simulink model "Li-ion_battery_vehicle"  (R2021a)
settings: Solver=VariableStepAuto  StartTime=0.0  StopTime=200  RelTol=1e-3
values from neighbouring files (symbols this model uses):
  air_density = 1.225    [matlabnew.mat]
  area = 5    [matlabnew.mat]
  braking_torque_to_pedal_force_ratio = -4    [matlabnew.mat]
  C1_LUT = [1913.6 4625.7 23306 10736 18036 12251 9022.9 12447 18872 40764 18721 33630 ... (21 elements, 7x3)]    [matlabnew.mat]
  Capacity_LUT = [28.0081 27.625 27.6392]    [matlabnew.mat]
  cell_Cp_heat = 810.5328    [matlabnew.mat]
  cell_mass = 1    [matlabnew.mat]
  drag_coefficient = 0.25    [matlabnew.mat]
  dt = 0.01    [matlabnew.mat]
  Em_LUT = [3.4966 3.5519 3.6183 3.7066 3.9131 4.0748 4.1923 3.5057 3.566 3.6337 3.7127 3.9259 ... (21 elements, 7x3)]    [matlabnew.mat]
  force_max_pedal = 500    [matlabnew.mat]
  gear_ratio = 6    [matlabnew.mat]
  gravity = 9.81    [matlabnew.mat]
  max_power = 50000    [matlabnew.mat]
  max_torque = 220    [matlabnew.mat]
  Qe_init = 15.6845    [matlabnew.mat]
  R0_LUT = [0.0117 0.011 0.0114 0.0107 0.0107 0.0113 0.0116 0.0085 0.0085 0.0087 0.0082 0.0083 ... (21 elements, 7x3)]    [matlabnew.mat]
  R1_LUT = [0.0109 0.0069 0.0047 0.0034 0.0033 0.0033 0.0028 0.0029 0.0024 0.0026 0.0016 0.0023 ... (21 elements, 7x3)]    [matlabnew.mat]
  rolling_res_ratio = 0.015    [matlabnew.mat]
  SOC_LUT = [0 0.1 0.25 0.5 0.75 0.9 1]    [matlabnew.mat]
  T_init = 293.15    [matlabnew.mat]
  Temperature_LUT = [278.15 293.15 313.15]    [matlabnew.mat]
  vehicle_mass = 1800    [matlabnew.mat]
  wheel_radius = 0.025    [matlabnew.mat]
undefined symbols (not defined in the file or in its folder): DiscIntNeverNeededParam, sigbuilder_block
libraries: fl_lib x57, fl_ps_legacy_lib x36, nesl_utility x13, LiBatteryElements_lib x4, ee_lib x2, simulink x2, simulink_extras x1, sim3dcameralib x1, sim3dlib x1, sim3dautolib x1
(part 2 of 2)

== system Li-ion_battery_vehicle/Vehicle Control/Max Power ==
  Vspd : Inport
  Abs : Abs
  Constant : Constant
  Math Function : Math  Operator=reciprocal  SignedPower=on  SaturateOnIntegerOverflow=on
  Prevent divide by zero : Switch  Criteria=u2 > Threshold  Threshold=1
  max_power : Gain  Gain=max_power
  Max Power : Outport  VectorParamsAs1DForOutWhenUnconnected=off
  wires:
  Prevent divide by zero/1 -> Math Function/1
  Constant/1 -> Prevent divide by zero/3
  Abs/1 -> Prevent divide by zero/2, Prevent divide by zero/1
  Math Function/1 -> max_power/1
  max_power/1 -> Max Power/1
  Vspd/1 -> Abs/1

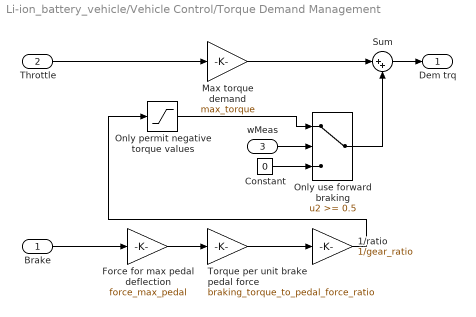
== system Li-ion_battery_vehicle/Vehicle Control/Torque Demand Management ==
  Brake : Inport
  Throttle : Inport  Port=2
  wMeas : Inport  Port=3
  1/ratio : Gain  Gain=1/gear_ratio
  Constant : Constant  Value=0  SampleTime=dt
  Force for max pedal deflection : Gain  Gain=force_max_pedal
  Max torque demand : Gain  Gain=max_torque
  Only permit negative torque values : Saturate  UpperLimit=-10  LowerLimit=-max_torque
  Only use forward braking : Switch  Threshold=0.5  InputSameDT=on
  Sum : Sum  Inputs=|++
  Torque per unit brake pedal force : Gain  Gain=braking_torque_to_pedal_force_ratio
  Dem trq : Outport  VectorParamsAs1DForOutWhenUnconnected=off
  wires:
  Max torque demand/1 -> Sum/1
  Brake/1 -> Force for max pedal deflection/1
  Sum/1 -> Dem trq/1
  Throttle/1 -> Max torque demand/1
  Torque per unit brake pedal force/1 -> 1/ratio/1
  1/ratio/1 -> Only permit negative torque values/1
  Force for max pedal deflection/1 -> Torque per unit brake pedal force/1
  wMeas/1 -> Only use forward braking/2
  Only use forward braking/1 -> Sum/2
  Constant/1 -> Only use forward braking/3
  Only permit negative torque values/1 -> Only use forward braking/1

== system Li-ion_battery_vehicle/Vehicle Control/regenerative braking  ==
  Inclin. : Inport
  " M " : Gain  Gain=vehicle_mass
  1/ratio : Gain  Gain=1/gear_ratio
  Wheel radius : Gain  Gain=wheel_radius
  Feedfwd trq : Outport  VectorParamsAs1DForOutWhenUnconnected=off
  wires:
  Inclin./1 -> " M "/1
  " M "/1 -> Wheel radius/1
  Wheel radius/1 -> 1/ratio/1  "Wheel torque"
  1/ratio/1 -> Feedfwd trq/1  "Motor torque"

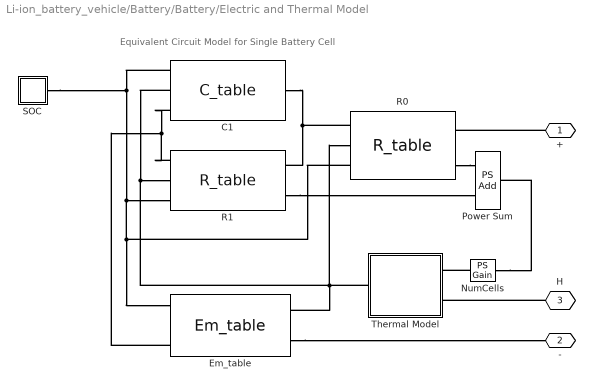
== system Li-ion_battery_vehicle/Battery/Battery/Electric and Thermal Model ==
  note: Equivalent Circuit Model for Single Battery Cell
  " SOC " : Subsystem
  C1 : LiBatteryElements_lib/C_table  C_Table=C1_LUT*Nparallel F  SOC_Table=SOC_LUT  Temp_Table=Temperature_LUT K  v0=0 V
      settings: SourceProductBaseCode=SS  InternalSimscapePortConfiguration="{\"Bottom\":[],\"Left\":[{\"id\":\"p\",\"label\":\"+\",\"type\":\"foundation.electrical.electrical\"},{\"id\":\"T\",\"label\":\"T\",\"type\":\"input\"},{\"id\":\"SOC\",\"label\":\"SOC\",\"type\":\"input\"}],\"Right\":[{\"id\":\"n\",\"label\":\"-\",\"type\":\"foundation.electrical.electrical\"}],\"Top\":[]}"
  Em_table : LiBatteryElements_lib/Em_table  C_Table=Capacity_LUT*Nparallel hr*A  Em_Table=Em_LUT V  SOC_Table=SOC_LUT  Temp_Table=Temperature_LUT K  Qinit=Qe_init*Nparallel hr*A
      settings: SourceProductBaseCode=SS  InternalSimscapePortConfiguration="{\"Bottom\":[],\"Left\":[{\"id\":\"p\",\"label\":\"+\",\"type\":\"foundation.electrical.electrical\"},{\"id\":\"C\",\"label\":\"C\",\"type\":\"output\"},{\"id\":\"SOC\",\"label\":\"SOC\",\"type\":\"output\"}],\"Right\":[{\"id\":\"n\",\"label\":\"-\",\"type\":\"foundation.electrical.electrical\"},{\"id\":\"T\",\"label\":\"T\",\"type\":\"input\"}],\"Top\":[]}"
  NumCells : fl_ps_legacy_lib/Legacy Physical Signals/Functions/PS Gain  gain=Nseries
  Power Sum : fl_ps_legacy_lib/Legacy Physical Signals/Functions/PS Add
      settings: SourceProductBaseCode=SS  InternalSimscapePortConfiguration="{\"Bottom\":[],\"Left\":[{\"id\":\"I1\",\"label\":\"\",\"type\":\"input\"},{\"id\":\"I2\",\"label\":\"\",\"type\":\"input\"}],\"Right\":[{\"id\":\"O\",\"label\":\"\",\"type\":\"output\"}],\"Top\":[]}"
  R0 : LiBatteryElements_lib/R_table  R_Table=R0_LUT/Nparallel Ohm  SOC_Table=SOC_LUT  Temp_Table=Temperature_LUT K
      settings: SourceProductBaseCode=SS  InternalSimscapePortConfiguration="{\"Bottom\":[],\"Left\":[{\"id\":\"p\",\"label\":\"+\",\"type\":\"foundation.electrical.electrical\"},{\"id\":\"T\",\"label\":\"T\",\"type\":\"input\"},{\"id\":\"SOC\",\"label\":\"SOC\",\"type\":\"input\"}],\"Right\":[{\"id\":\"n\",\"label\":\"-\",\"type\":\"foundation.electrical.electrical\"},{\"id\":\"pow\",\"label\":\"POW\",\"type\":\"output\"}],\"Top\":[]}"
  R1 : LiBatteryElements_lib/R_table  R_Table=R1_LUT/Nparallel Ohm  SOC_Table=SOC_LUT  Temp_Table=Temperature_LUT K
      settings: SourceProductBaseCode=SS  InternalSimscapePortConfiguration="{\"Bottom\":[],\"Left\":[{\"id\":\"p\",\"label\":\"+\",\"type\":\"foundation.electrical.electrical\"},{\"id\":\"T\",\"label\":\"T\",\"type\":\"input\"},{\"id\":\"SOC\",\"label\":\"SOC\",\"type\":\"input\"}],\"Right\":[{\"id\":\"n\",\"label\":\"-\",\"type\":\"foundation.electrical.electrical\"},{\"id\":\"pow\",\"label\":\"POW\",\"type\":\"output\"}],\"Top\":[]}"
  Thermal Model : Subsystem
  + : PMIOPort  Side=Right
  - : PMIOPort  Port=2  Side=Right
  H : PMIOPort  Tag=PMCPort  Port=3  Side=Left
  connections:
  NumCells/LConn1 -- Power Sum/RConn1
  +/RConn1 -- R0/RConn1
  C1/LConn2 -- Thermal Model/RConn1 -- Em_table/RConn2 -- R0/LConn2 -- R1/LConn2
  Em_table/LConn1 -- R1/LConn1 -- C1/LConn1
  R1/RConn2 -- Power Sum/LConn2
  R0/RConn2 -- Power Sum/LConn1
  C1/RConn1 -- R1/RConn1 -- R0/LConn1
  Em_table/RConn1 -- -/RConn1
  R0/LConn3 -- Em_table/LConn3 -- " SOC "/LConn1 -- C1/LConn3 -- R1/LConn3
  NumCells/RConn1 -- Thermal Model/LConn1
  H/RConn1 -- Thermal Model/LConn2

== system Li-ion_battery_vehicle/Battery/Cooling System/Heat Exch. Characteristic ==
  Characteristic : Subsystem
  Heat Flow Source : fl_lib/Thermal/Thermal Sources/Controlled Heat Flow Rate Source
  Mass Flow Rate & Thermal Flux Sensor (TL) : fl_lib/Thermal Liquid/Sensors/Mass & Energy Flow Rate Sensor (TL)
      settings: SourceProductBaseCode=SS  InternalSimscapePortConfiguration="{\"Bottom\":[],\"Left\":[{\"id\":\"A\",\"label\":\"A\",\"type\":\"foundation.thermal_liquid.thermal_liquid\"}],\"Right\":[{\"id\":\"B\",\"label\":\"B\",\"type\":\"foundation.thermal_liquid.thermal_liquid\"},{\"id\":\"M\",\"label\":\"M\",\"type\":\"output\"},{\"id\":\"PHI\",\"label\":\"Phi\",\"type\":\"output\"}],\"Top\":[]}"
  Temperature Sensor : fl_lib/Thermal/Thermal Sensors/Temperature Sensor
  ThRef : fl_lib/Thermal/Thermal Elements/Thermal Reference
  Henv : PMIOPort  Side=Right
  Hp : PMIOPort  Port=2  Side=Left
  B : PMIOPort  Port=3  Side=Right
  Phi : PMIOPort  Port=4  Side=Right
  A : PMIOPort  Port=5  Side=Left
  T in : PMIOPort  Port=6  Side=Left
  connections:
  A/RConn1 -- Mass Flow Rate & Thermal Flux Sensor (TL)/LConn1
  Temperature Sensor/LConn1 -- Henv/RConn1 -- Heat Flow Source/RConn2
  ThRef/LConn1 -- Temperature Sensor/RConn1
  Heat Flow Source/LConn1 -- Hp/RConn1
  Mass Flow Rate & Thermal Flux Sensor (TL)/RConn1 -- B/RConn1
  Mass Flow Rate & Thermal Flux Sensor (TL)/RConn3 -- Phi/RConn1
  Mass Flow Rate & Thermal Flux Sensor (TL)/RConn2 -- Characteristic/RConn1
  T in/RConn1 -- Characteristic/RConn2
  Temperature Sensor/RConn2 -- Characteristic/RConn3
  Characteristic/LConn1 -- Heat Flow Source/RConn1

== system Li-ion_battery_vehicle/Battery/Cooling System/Sensing Temperature ==
  Pressure & Temperature Sensor (TL) : fl_lib/Thermal Liquid/Sensors/Pressure & Temperature Sensor (TL)
      settings: SourceProductBaseCode=SS  InternalSimscapePortConfiguration="{\"Bottom\":[],\"Left\":[{\"id\":\"A\",\"label\":\"A\",\"type\":\"foundation.thermal_liquid.thermal_liquid\"}],\"Right\":[{\"id\":\"B\",\"label\":\"B\",\"type\":\"foundation.thermal_liquid.thermal_liquid\"},{\"id\":\"P\",\"label\":\"P\",\"type\":\"output\"},{\"id\":\"T\",\"label\":\"T\",\"type\":\"output\"}],\"Top\":[]}"
  TLRef : fl_lib/Thermal Liquid/Elements/Absolute Reference (TL)
      settings: SourceProductBaseCode=SS
  T : PMIOPort  Side=Right
  A : PMIOPort  Port=2  Side=Left
  connections:
  Pressure & Temperature Sensor (TL)/RConn3 -- T/RConn1
  TLRef/LConn1 -- Pressure & Temperature Sensor (TL)/RConn1
  A/RConn1 -- Pressure & Temperature Sensor (TL)/LConn1

== system Li-ion_battery_vehicle/Battery/DC-DC Converter/Sensing Battery Quantities ==
  Battery Voltage : nesl_utility/PS-Simulink Converter  PhysicalDomain=network_engine_domain  SubClassName=ps_output  LeftPortType=input  RightPortType=output  PseudoPeriodic=off  Frequencies=[]  Unit=V  AffineConversion=off
      settings: SourceProductBaseCode=PW,SS
  Current Sensor : fl_lib/Electrical/Electrical Sensors/Current Sensor
  PS-Simulink Converter1 : nesl_utility/PS-Simulink Converter  PhysicalDomain=network_engine_domain  SubClassName=ps_output  LeftPortType=input  RightPortType=output  PseudoPeriodic=off  Frequencies=[]  Unit=A  AffineConversion=off
      settings: SourceProductBaseCode=PW,SS
  Voltage Sensor : fl_lib/Electrical/Electrical Sensors/Voltage Sensor
  +1 : PMIOPort  Side=Right
  - : PMIOPort  Port=2  Side=Left
  +2 : PMIOPort  Port=3  Side=Right
  tag scope: iBat=global, vBat=global
  wires:
  Battery Voltage/1 -> [vBat]
  PS-Simulink Converter1/1 -> [iBat]
  connections:
  Voltage Sensor/RConn2 -- -/RConn1
  Voltage Sensor/LConn1 -- Current Sensor/LConn1 -- +1/RConn1
  Voltage Sensor/RConn1 -- Battery Voltage/LConn1
  Current Sensor/RConn2 -- +2/RConn1
  Current Sensor/RConn1 -- PS-Simulink Converter1/LConn1

== system Li-ion_battery_vehicle/PMSM Drive/Heat Exch. Characteristic/Characteristic ==
  PS Product : fl_ps_legacy_lib/Legacy Physical Signals/Functions/PS Product
      settings: SourceProductBaseCode=SS
  PS Subtract : fl_ps_legacy_lib/Legacy Physical Signals/Functions/PS Subtract
      settings: SourceProductBaseCode=SS
  Specific dissipation (J/s/K) : fl_ps_legacy_lib/Legacy Physical Signals/Lookup Tables/PS Lookup Table (1D)  x="[0 0.2 0.4  0.7  1 1.2  1.4  2.5 ]"  f=100 * [0 0.5 0.75 0.92 1 1.02 1.03 1.04]  interp_method=1  extrap_method=1
      settings: SourceProductBaseCode=SS  InternalSimscapePortConfiguration="{\"Bottom\":[],\"Left\":[{\"id\":\"I\",\"label\":\"x\",\"type\":\"input\"}],\"Right\":[{\"id\":\"O\",\"label\":\"f\",\"type\":\"output\"}],\"Top\":[]}"
  Specific dissipation (J/s/K) per unit mass flow rate : fl_ps_legacy_lib/Legacy Physical Signals/Functions/PS Gain  gain=100
  Mass Flow : PMIOPort  Side=Left
  Temp Inlet : PMIOPort  Port=2  Side=Left
  Temp Motor : PMIOPort  Port=3  Side=Left
  Q : PMIOPort  Port=4  Side=Right
  connections:
  PS Subtract/RConn1 -- PS Product/LConn1
  Specific dissipation (J/s/K)/RConn1 -- PS Product/LConn2
  Temp Motor/RConn1 -- PS Subtract/LConn1
  PS Subtract/LConn2 -- Temp Inlet/RConn1
  PS Product/RConn1 -- Q/RConn1
  Mass Flow/RConn1 -- Specific dissipation (J/s/K) per unit mass flow rate/LConn1
  Specific dissipation (J/s/K) per unit mass flow rate/RConn1 -- Specific dissipation (J/s/K)/LConn1

== system Li-ion_battery_vehicle/Vehicle Dynamics/Brake Torque/Smooth Sign ==
  1 : fl_lib/Physical Signals/Sources/PS Constant  constant=1
  2 : fl_ps_legacy_lib/Legacy Physical Signals/Functions/PS Gain  gain=2
  exp(2x) : fl_ps_legacy_lib/Legacy Physical Signals/Functions/PS Math Function  fcn_choice=3
      settings: SourceProductBaseCode=SS  InternalSimscapePortConfiguration="{\"Bottom\":[],\"Left\":[{\"id\":\"I\",\"label\":\"\",\"type\":\"input\"}],\"Right\":[{\"id\":\"O\",\"label\":\"\",\"type\":\"output\"}],\"Top\":[]}"
  exp(2x)+1 : fl_ps_legacy_lib/Legacy Physical Signals/Functions/PS Add
      settings: SourceProductBaseCode=SS  InternalSimscapePortConfiguration="{\"Bottom\":[],\"Left\":[{\"id\":\"I1\",\"label\":\"\",\"type\":\"input\"},{\"id\":\"I2\",\"label\":\"\",\"type\":\"input\"}],\"Right\":[{\"id\":\"O\",\"label\":\"\",\"type\":\"output\"}],\"Top\":[]}"
  exp(2x)-1 : fl_ps_legacy_lib/Legacy Physical Signals/Functions/PS Subtract
      settings: SourceProductBaseCode=SS
  tanh(x) : fl_ps_legacy_lib/Legacy Physical Signals/Functions/PS Divide
      settings: SourceProductBaseCode=SS  InternalSimscapePortConfiguration="{\"Bottom\":[],\"Left\":[{\"id\":\"I1\",\"label\":\"\",\"type\":\"input\"},{\"id\":\"I2\",\"label\":\"\",\"type\":\"input\"}],\"Right\":[{\"id\":\"O\",\"label\":\"\",\"type\":\"output\"}],\"Top\":[]}"
  x : PMIOPort  Side=Left
  y : PMIOPort  Port=2  Side=Right
  connections:
  y/RConn1 -- tanh(x)/RConn1
  x/RConn1 -- 2/LConn1
  exp(2x)-1/RConn1 -- tanh(x)/LConn1
  exp(2x)+1/RConn1 -- tanh(x)/LConn2
  exp(2x)+1/LConn2 -- exp(2x)-1/LConn1 -- exp(2x)/RConn1
  2/RConn1 -- exp(2x)/LConn1
  exp(2x)-1/LConn2 -- exp(2x)+1/LConn1 -- 1/RConn1

== system Li-ion_battery_vehicle/Vehicle Dynamics/Drag and Gravity/Smooth Step ==
  1 : fl_lib/Physical Signals/Sources/PS Constant  constant=1
  2 : fl_ps_legacy_lib/Legacy Physical Signals/Functions/PS Gain  gain=2
  exp(2x) : fl_ps_legacy_lib/Legacy Physical Signals/Functions/PS Math Function  fcn_choice=3
      settings: SourceProductBaseCode=SS  InternalSimscapePortConfiguration="{\"Bottom\":[],\"Left\":[{\"id\":\"I\",\"label\":\"\",\"type\":\"input\"}],\"Right\":[{\"id\":\"O\",\"label\":\"\",\"type\":\"output\"}],\"Top\":[]}"
  exp(2x)+1 : fl_ps_legacy_lib/Legacy Physical Signals/Functions/PS Add
      settings: SourceProductBaseCode=SS  InternalSimscapePortConfiguration="{\"Bottom\":[],\"Left\":[{\"id\":\"I1\",\"label\":\"\",\"type\":\"input\"},{\"id\":\"I2\",\"label\":\"\",\"type\":\"input\"}],\"Right\":[{\"id\":\"O\",\"label\":\"\",\"type\":\"output\"}],\"Top\":[]}"
  exp(2x)-1 : fl_ps_legacy_lib/Legacy Physical Signals/Functions/PS Subtract
      settings: SourceProductBaseCode=SS
  tanh(x) : fl_ps_legacy_lib/Legacy Physical Signals/Functions/PS Divide
      settings: SourceProductBaseCode=SS  InternalSimscapePortConfiguration="{\"Bottom\":[],\"Left\":[{\"id\":\"I1\",\"label\":\"\",\"type\":\"input\"},{\"id\":\"I2\",\"label\":\"\",\"type\":\"input\"}],\"Right\":[{\"id\":\"O\",\"label\":\"\",\"type\":\"output\"}],\"Top\":[]}"
  x : PMIOPort  Side=Left
  y : PMIOPort  Port=2  Side=Right
  connections:
  y/RConn1 -- tanh(x)/RConn1
  x/RConn1 -- 2/LConn1
  exp(2x)-1/RConn1 -- tanh(x)/LConn1
  exp(2x)+1/RConn1 -- tanh(x)/LConn2
  exp(2x)+1/LConn2 -- exp(2x)-1/LConn1 -- exp(2x)/RConn1
  2/RConn1 -- exp(2x)/LConn1
  exp(2x)-1/LConn2 -- exp(2x)+1/LConn1 -- 1/RConn1

== system Li-ion_battery_vehicle/Vehicle Control/Cruise Control/Capture speed ==
  In1 : Inport
  Trigger : TriggerPort  VariantControl=Variant
  Out1 : Outport  VectorParamsAs1DForOutWhenUnconnected=off
  wires:
  In1/1 -> Out1/1

== system Li-ion_battery_vehicle/Vehicle Control/Cruise Control/Speed Controller ==
  wRef : Inport
  wMeas : Inport  Port=2
  Add : Sum  Inputs=|+-
  Add1 : Sum
  Discrete-Time Integrator : DiscreteIntegrator  gainval=Ki  SampleTime=ts  LimitOutput=on  UpperSaturationLimit=trqMax  LowerSaturationLimit=-trqMax  ICPrevOutput=DiscIntNeverNeededParam  ICPrevScaledInput=DiscIntNeverNeededParam
  Kp : Gain  Gain=Kp
  trqRef : Outport  VectorParamsAs1DForOutWhenUnconnected=off
  wires:
  wRef/1 -> Add/1
  Kp/1 -> Add1/1
  Discrete-Time Integrator/1 -> Add1/2
  wMeas/1 -> Add/2
  Add1/1 -> trqRef/1
  Add/1 -> Kp/1, Discrete-Time Integrator/1

== system Li-ion_battery_vehicle/Battery/Battery/Electric and Thermal Model/ SOC  ==
  PS-Simulink Converter1 : nesl_utility/PS-Simulink Converter  PhysicalDomain=network_engine_domain  SubClassName=ps_output  LeftPortType=input  RightPortType=output  PseudoPeriodic=off  Frequencies=[]  Unit=1  AffineConversion=off
      settings: SourceProductBaseCode=PW,SS
  PS : PMIOPort  Side=Left
  tag scope: SOC=global
  wires:
  PS-Simulink Converter1/1 -> [SOC]
  connections:
  PS/RConn1 -- PS-Simulink Converter1/LConn1

== system Li-ion_battery_vehicle/Battery/Battery/Electric and Thermal Model/Thermal Model ==
  Battery Thermal Mass : fl_lib/Thermal/Thermal Elements/Thermal Mass  mass=cell_mass*Nseries*Nparallel kg  sp_heat=cell_Cp_heat J/kg/K  T_specify=on  T_priority=High  T=T_init K  T_nominal_specify=off  T_nominal_unit=K  T_nominal_value=1  Q_specify=off  Q_priority=High  Q=0 J/s  Q_nominal_specify=off  Q_nominal_unit=J/s  Q_nominal_value=1
  Heat Flow Source : fl_lib/Thermal/Thermal Sources/Controlled Heat Flow Rate Source
  Ideal Temperature Sensor : fl_lib/Thermal/Thermal Sensors/Temperature Sensor
  ThRef1 : fl_lib/Thermal/Thermal Elements/Thermal Reference
  ThRef2 : fl_lib/Thermal/Thermal Elements/Thermal Reference
  PlossTotal : PMIOPort  Tag=PMCPort  Side=Left
  T : PMIOPort  Tag=PMCPort  Port=2  Side=Right
  H : PMIOPort  Tag=PMCPort  Port=3  Side=Left
  connections:
  ThRef2/LConn1 -- Ideal Temperature Sensor/RConn1
  Ideal Temperature Sensor/RConn2 -- T/RConn1
  ThRef1/LConn1 -- Heat Flow Source/RConn2
  Ideal Temperature Sensor/LConn1 -- H/RConn1 -- Battery Thermal Mass/LConn1 -- Heat Flow Source/LConn1
  Heat Flow Source/RConn1 -- PlossTotal/RConn1

== system Li-ion_battery_vehicle/Battery/Cooling System/Heat Exch. Characteristic/Characteristic ==
  PS Product : fl_ps_legacy_lib/Legacy Physical Signals/Functions/PS Product
      settings: SourceProductBaseCode=SS
  PS Subtract : fl_ps_legacy_lib/Legacy Physical Signals/Functions/PS Subtract
      settings: SourceProductBaseCode=SS
  Specific dissipation (J/s/K) per unit mass flow rate : fl_ps_legacy_lib/Legacy Physical Signals/Functions/PS Gain  gain=100
  M : PMIOPort  Side=Right
  T in : PMIOPort  Port=2  Side=Right
  T Env : PMIOPort  Port=3  Side=Right
  Q : PMIOPort  Port=4  Side=Left
  connections:
  T Env/RConn1 -- PS Subtract/LConn1
  PS Product/RConn1 -- Q/RConn1
  PS Subtract/RConn1 -- PS Product/LConn1
  T in/RConn1 -- PS Subtract/LConn2
  M/RConn1 -- Specific dissipation (J/s/K) per unit mass flow rate/LConn1
  PS Product/LConn2 -- Specific dissipation (J/s/K) per unit mass flow rate/RConn1
